simulink model "generic_mass_SoC_mu"  (R2025a)
settings: Solver=ode45  StartTime=0.0  StopTime=12  RelTol=1e-3  EnableMultiTasking=on
values from neighbouring files (symbols this model uses):
  Battery =     [Battery_A123_Pack_204s2p_Final.mat]
  cs_tyre = 2.0e5    (= 200000)    [mu_estimator_parameters.m]
  dOCV_dSoC = gradient(OCV, SoC_bp)    [SoCOcv.m]
  dR0 = gradient(R0, SoC_L)    [SoCOcv.m]
  eps_vx = 0.5    [mu_estimator_parameters.m]
  fz_max = 6000    [mu_estimator_parameters.m]
  fz_min = 300    [mu_estimator_parameters.m]
  h_cg = 0.55    [mu_estimator_parameters.m]
  lf = 1.214    [mu_estimator_parameters.m]
  lr = 1.505    [mu_estimator_parameters.m]
  r0 = 0.344    [mu_estimator_parameters.m]
  re_max = 0.33    [mu_estimator_parameters.m]
  re_min = 0.28    [mu_estimator_parameters.m]
  SoC_bp = Table_SoCvsOCV.LUT.SoC_percent    [SoCOcv.m]
  SoC_L = Battery.SOC_LUT    [SoCOcv.m]
  Table_SoCvsOCV = load("SoC_to_Voltage_LUT_10000-GON.mat")    [SoCOcv.m]
  tw_f = 1.571    [mu_estimator_parameters.m]
  tw_r = 1.581    [mu_estimator_parameters.m]
undefined symbols (not defined in the file or in its folder): DiscIntNeverNeededParam, Init_SoC
libraries: CarMaker4SL x41, simulink x1
(part 4 of 4)

== matlab function generic_mass_SoC_mu/CarMaker/EKF ==
  settings: updateMethod=DISCRETE
  data: I input; soc_hat output; UL_meas input; Uoc input; R0_est input; R0nom input; R1 input; C1 input; dUoc_dSoc input; reset input; u1_hat output; ul_hat output; innov output; K_out output; P_out output; Qcap_est input; Qnom input
function [soc_hat, u1_hat, ul_hat, innov, K_out, P_out] = ...
    soc_ekf_paper_1rc(I, UL_meas, Uoc, R0_est, R0nom, R1, C1, dUoc_dSoc, reset, Qcap_est,Qnom)

    persistent x_hat P initialized

    Dt   = 0.01;
    Qnom = 3.6*Qnom;
    Qcap_est = Qcap_est*3600;
    

    Rekf = 1e-1;

    if isempty(initialized) || reset
        x_hat = [0.8;
                 0.0];

        P = [1e-6, 0;
             0,    1e-6];

        initialized = true;
    end

    
    if Qcap_est > 0
        Q0 = Qcap_est;
    else
        Q0 = Qnom;
    end

    
    if R0_est > 1e-3
        R0 = R0_est;
    else
        R0 = R0nom;
    end

    tau1 = R1 * C1;
    a1 = exp(-Dt / tau1);

    A = [1,  0;
         0, a1];

    B = [-Dt / Q0;
         R1 * (1 - exp(-Dt / tau1))];

    sigma_I2 = 1e-1;
    Q_input  = (B * B.') * sigma_I2;

    Q_base = [1e-8, 0;
              0,    1e-8];

    Qekf = Q_base + Q_input;

    % (1) State prediction
    x_pred = A * x_hat + B * I;

    % (2) Covariance prediction
    P_pred = A * P * A.' + Qekf;

    % (3) Measurement Jacobian
    C = [dUoc_dSoc, -1];

    % (4) Predicted output
    ul_hat = Uoc - R0 * I - x_pred(2);

    % (5) Kalman gain
    S = C * P_pred * C.' + Rekf;
    K = (P_pred * C.') / S;

    % (6) State update
    innov = UL_meas - ul_hat;
    x_hat = x_pred + K * innov;

    % (7) Covariance update
    I2 = eye(2);
    P = (I2 - K * C) * P_pred;

    % Outputs
    soc_hat = x_hat(1);
    u1_hat  = x_hat(2);
    K_out   = K;
    P_out   = P;
end

== matlab function generic_mass_SoC_mu/CarMaker/RC network subsystem/MATLAB Function ==
  data: I input; y output; R1 input; C1 input; V1 input
function y = fcn(I,R1,C1,V1)

y = -V1/(R1*C1)+I/C1;

== matlab function generic_mass_SoC_mu/CarMaker/Mass Estimator ==
  settings: updateMethod=DISCRETE
  data: y input; phi input; lambda input; m_hat output; t input; ax input
function m_hat = mass_rls(y, phi, lambda, t, ax)
    persistent theta P initialized t_start est_active done
    if isempty(initialized)
        theta = 1/2200;
        P = 1e6;
        t_start = 0;
        est_active = false;
        done = false;
        initialized = true;
    end
    theta_min = 1/3000;
    theta_max = 1/1500;
   
    if ~done && ~est_active && abs(ax) > 0.5
        est_active = true;
        t_start = t;
    end
   
    if est_active
        if (t - t_start) <= 10
            eps = y - phi * theta;
            L = (P * phi) / (lambda + phi * P * phi);
            theta = theta + L * eps;
            P = (P * (1 - L * phi)) / lambda;
            if theta < theta_min
                theta = theta_min;
            elseif theta > theta_max
                theta = theta_max;
            end
        else
            est_active = false;
            done = true;
        end
    end
    m_hat = 1 / theta;
end

== matlab function generic_mass_SoC_mu/CarMaker/MATLAB Function2 ==
  data: ax input; y output; beta input
function y = compute_y(ax,beta) 
g=9.81; 
f=0.015; 
delta=1; 
y = delta*ax + g*f + g*sin(beta);
